simulink model "Ex6_1_1_PID"  (R2016a)
settings: Solver=VariableStepAuto  StartTime=0.0  StopTime=20  RelTol=1e-3
settings Model: Creator=mende  LastModifiedBy=mende

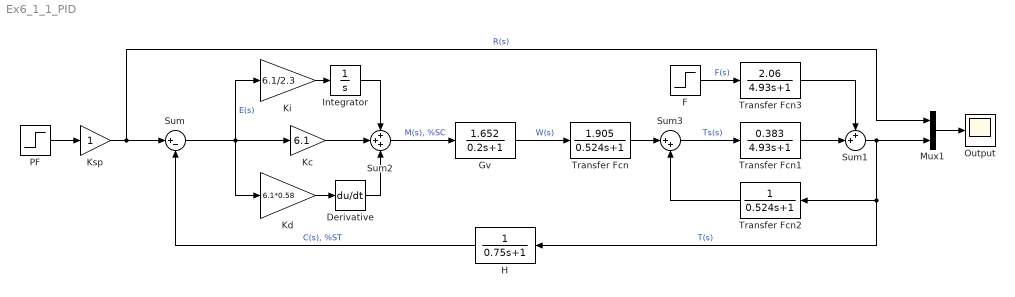
== system Ex6_1_1_PID ==
  Derivative : Derivative
  F : Step  SampleTime=0
  Gv : TransferFcn  Numerator=[1.652]  Denominator=[0.2 1]
  H : TransferFcn  Denominator=[0.75 1]
  Integrator : Integrator
  Kc : Gain  Gain=6.1
  Kd : Gain  Gain=6.1*0.58
  Ki : Gain  Gain=6.1/2.3
  Ksp : Gain
  Mux1 : Mux  Inputs=2
  Output : Scope
  PF : Step  SampleTime=0
  Sum : Sum  Inputs=|+-
  Sum1 : Sum  Inputs=++|
  Sum2 : Sum  Inputs=+++
  Sum3 : Sum  Inputs=|++
  Transfer Fcn : TransferFcn  Numerator=[1.905]  Denominator=[0.524 1]
  Transfer Fcn1 : TransferFcn  Numerator=[0.383]  Denominator=[4.93 1]
  Transfer Fcn2 : TransferFcn  Denominator=[0.524 1]
  Transfer Fcn3 : TransferFcn  Numerator=[2.06]  Denominator=[4.93 1]
  wires:
  Ksp/1 -> Sum/1, Mux1/1  "R(s)"
  Sum/1 -> Ki/1, Kc/1, Kd/1  "E(s)"
  Gv/1 -> Transfer Fcn/1  "W(s)"
  H/1 -> Sum/2  "C(s), %ST"
  Sum1/1 -> Mux1/2, H/1, Transfer Fcn2/1  "T(s)"
  Mux1/1 -> Output/1
  PF/1 -> Ksp/1
  Sum2/1 -> Gv/1  "M(s), %SC"
  Kc/1 -> Sum2/2
  Kd/1 -> Derivative/1
  Ki/1 -> Integrator/1
  Integrator/1 -> Sum2/1
  Derivative/1 -> Sum2/3
  Transfer Fcn1/1 -> Sum1/2
  F/1 -> Transfer Fcn3/1  "F(s)"
  Transfer Fcn3/1 -> Sum1/1
  Transfer Fcn2/1 -> Sum3/2
  Transfer Fcn/1 -> Sum3/1
  Sum3/1 -> Transfer Fcn1/1  "Ts(s)"
